simulink model "Prob4"  (R2020b)
settings: Solver=VariableStepAuto  StartTime=0.0  StopTime=10.0  RelTol=1e-3
settings Model: Creator=stkaravind  LastModifiedBy=stkaravind

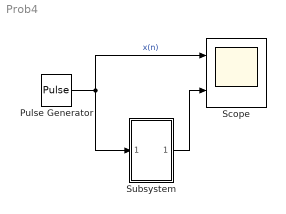
== system Prob4 ==
  Pulse Generator : DiscretePulseGenerator  PulseType=Time based  Period=10  PulseWidth=5
  Scope : Scope  NumInputPorts=2
  Subsystem : Subsystem
  wires:
  Pulse Generator/1 -> Scope/1, Subsystem/1(x(n))  "x(n)"
  Subsystem/1(y(n)) -> Scope/2

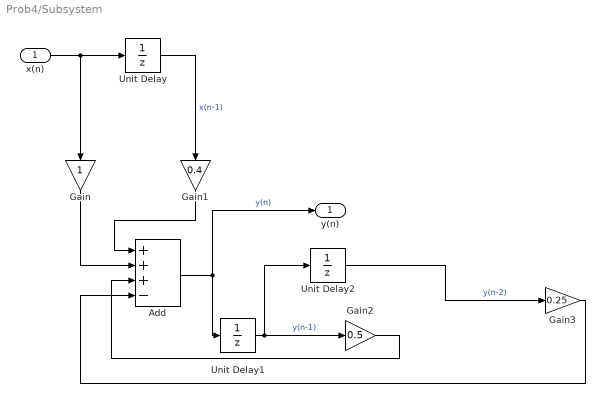
== system Prob4/Subsystem ==
  x(n) : Inport
  Add : Sum  Inputs=+++-
  Gain : Gain
  Gain1 : Gain  Gain=0.4
  Gain2 : Gain  Gain=0.5
  Gain3 : Gain  Gain=0.25
  Unit Delay : UnitDelay  SampleTime=-1  HasFrameUpgradeWarning=on
  Unit Delay1 : UnitDelay  SampleTime=-1  HasFrameUpgradeWarning=on
  Unit Delay2 : UnitDelay  SampleTime=-1  HasFrameUpgradeWarning=on
  y(n) : Outport
  wires:
  x(n)/1 -> Gain/1, Unit Delay/1
  Gain1/1 -> Add/1
  Gain3/1 -> Add/4
  Unit Delay/1 -> Gain1/1  "x(n-1)"
  Gain2/1 -> Add/3
  Unit Delay1/1 -> Unit Delay2/1, Gain2/1  "y(n-1)"
  Gain/1 -> Add/2
  Add/1 -> y(n)/1, Unit Delay1/1  "y(n)"
  Unit Delay2/1 -> Gain3/1  "y(n-2)"
